simulink model "sim_tase_2025_att_ctrl"  (R2020a)
settings: Solver=ode4  StartTime=0.0  StopTime=30.0  FixedStep=0.01  RelTol=1e-3
values from neighbouring files (symbols this model uses):
  alfa_i_init = zeros(3, NF)    [init_tase_2025_att_ctrl.m]
  beta_ij_init = zeros(3, NF)    [init_tase_2025_att_ctrl.m]
  c1 = 2.5    [init_tase_2025_att_ctrl.m]
  c1_diff_sigma_bar_w = diag([12; 12; 12])    [init_tase_2025_att_ctrl.m]
  c1_diff_ui = diag([25; 30; 20])    [init_tase_2025_att_ctrl.m]
  c2 = 2.0    (= 2)    [init_tase_2025_att_ctrl.m]
  c2_diff_sigma_bar_w = diag([12; 12; 12])    [init_tase_2025_att_ctrl.m]
  c2_diff_ui = diag([50; 50; 10])    [init_tase_2025_att_ctrl.m]
  c3_diff_sigma_bar_w = diag([15; 15; 15])    [init_tase_2025_att_ctrl.m]
  c3_diff_ui = diag([15; 15; 10])    [init_tase_2025_att_ctrl.m]
  dw_aa_t = 0.2 * ones(3, 5) + ( 1.0 - 0.2 ) * rand(3, 5)    [init_tase_2025_att_ctrl.m]
  dw_ff_t = [ 0.4 * ones(1, 5) + ( 1.0 - 0.4 ) * rand(1, 5);                      0.4 * ones(1, 5) + ( 1.0 - 0.4 ) * rand(1, 5);                      0.2 * ones(1, 5) + ( 0.6 - 0.2 ) * rand(1, 5) ]    [init_tase_2025_att_ctrl.m]
  dw_phi_t = ( - pi / 2 ) * ones(3, 5) + ( pi / 2 - ( - pi / 2 ) ) * rand(3, 5)    [init_tase_2025_att_ctrl.m]
  dwci_init = zeros(3,5)    [init_tase_2025_att_ctrl.m]
  err_wi_init = zeros(3, NF)    [init_tase_2025_att_ctrl.m]
  eta_1_ij_init = zeros(3, NF)    [init_tase_2025_att_ctrl.m]
  eta_2_ij_init = zeros(3, NF)    [init_tase_2025_att_ctrl.m]
  h1w = diag([20.0; 20.0; 20.0])    [init_tase_2025_att_ctrl.m]
  h2w = diag([30.0; 35.0; 35.0])    [init_tase_2025_att_ctrl.m]
  h3w = diag([30.0; 25.0; 30.0])    [init_tase_2025_att_ctrl.m]
  Ji = zeros(3,3,NF)    [init_tase_2025_att_ctrl.m]
  k_1_ij_hat_init = zeros(3, NF)    [init_tase_2025_att_ctrl.m]
  k_1_ij_init = zeros(3, NF)    [init_tase_2025_att_ctrl.m]
  k_1_ij_lower = zeros(3, NF)    [init_tase_2025_att_ctrl.m]
  k_1_ij_upper = zeros(3, NF)    [init_tase_2025_att_ctrl.m]
  k_2_ij_init = zeros(3, NF)    [init_tase_2025_att_ctrl.m]
  k_2_ij_lower = zeros(3, NF)    [init_tase_2025_att_ctrl.m]
  k_2_ij_upper = zeros(3, NF)    [init_tase_2025_att_ctrl.m]
  Lamd_diff_sigma_bar_w = 0.8    [init_tase_2025_att_ctrl.m]
  Lamd_diff_ui = 0.8    [init_tase_2025_att_ctrl.m]
  mu1 = 0.2    [init_tase_2025_att_ctrl.m]
  mu2 = 0.2    [init_tase_2025_att_ctrl.m]
  mu_d_w = 100    [init_tase_2025_att_ctrl.m]
  phi_ij_init = ones(3, NF)    [init_tase_2025_att_ctrl.m]
  pos0 = zeros(3, 1)    [init_tase_2025_att_ctrl.m]
  PZ0 = P0(3)    [init_tase_2025_att_ctrl.m]
  PZ1 = 10    [init_tase_2025_att_ctrl.m]
  q_ij_hat_init = zeros(3, NF)    [init_tase_2025_att_ctrl.m]
  Qci_init = repmat([1;0;0;0],1,NF)    [init_tase_2025_att_ctrl.m]
  R0 = 4    [init_tase_2025_att_ctrl.m]
  R1 = 8    [init_tase_2025_att_ctrl.m]
  Rci_init = zeros(3,3,NF)    [init_tase_2025_att_ctrl.m]
  Ri_init = zeros(3,3,NF)    [init_tase_2025_att_ctrl.m]
  Rx2 = 10    [init_tase_2025_att_ctrl.m]
  Ry2 = 6    [init_tase_2025_att_ctrl.m]
  Rz2 = 4    [init_tase_2025_att_ctrl.m]
  T0 = 0    [init_tase_2025_att_ctrl.m]
  T1 = tseq1    (= 10)    [init_tase_2025_att_ctrl.m]
  T2 = tseq1 + tseq12 + tseq2    (= 30)    [init_tase_2025_att_ctrl.m]
  T_ij = repmat([60.0; 60.0; 60.0], 1, NF)    [init_tase_2025_att_ctrl.m]
  ui_init = zeros(3,NF)    [init_tase_2025_att_ctrl.m]
  vel0 = zeros(3, 1)    [init_tase_2025_att_ctrl.m]
  wci_init = zeros(3,5)    [init_tase_2025_att_ctrl.m]
  zeta_diff_sigma_bar_w = 0.3    [init_tase_2025_att_ctrl.m]
  zeta_diff_ui = 0.05    [init_tase_2025_att_ctrl.m]
undefined symbols (not defined in the file or in its folder): cal_frac_squ, p_alfaw1, p_alfaw2, q_alfaw1, q_alfaw2, Qei_init, Qi_init, Rei_init, V_Phi_Rei_init, wei_init, wi_init
(part 5 of 5)

== matlab function sim_tase_2025_att_ctrl/generate angular rate disturbance agent 3 ==
  data: dw_3 output; dw_aa_t input; dw_ff_t input; dw_phi_t input; t input
function dw_3 = fcn(dw_aa_t, dw_ff_t, dw_phi_t, t)
%%%% 姿态动力学方程中的扰动项设置
epsil_t = zeros(3, 1);

for kk = 1:5
    epsil_t = epsil_t + dw_aa_t(:, kk) .* sin( 2 * pi * dw_ff_t(:, kk) * t + dw_phi_t(:, kk) );
end

dw_3 = [ epsil_t(1) + 1.6 * sin( 0.2 * t ) + 2.0 * cos( 0.3 * t ) + 1.4 * sin( 0.5 * t ) ...
                + 4 * exp( -0.1 * t ) * sin( 0.5 * t ) + 3 / ( 1 + exp( -0.2 * ( t - 15 ) ) ); ...
                epsil_t(2) + 1.2 * sin( 0.1 * t ) + 3 * cos( 0.2 * t ) + 0.8 * sin( 0.4 * t ) ...
                + 2 * exp( -0.15 * t ) * cos( 0.6 * t ) + 3 / ( 1 + exp( -0.3 * ( t - 25 ) ) ); ...
                epsil_t(3) + 1.8 * sin( 0.1 * t ) + 1.6 * sin( 0.2 * t ) + 1.6 * cos( 0.3 * t ) ...
                + 4 * exp( -0.05 * t ) * sin( 0.4 * t + pi / 4 ) + 3 / ( 1 + exp( -0.5 * ( t - 20 ) ) ) ];

== matlab function sim_tase_2025_att_ctrl/generate angular rate disturbance agent 4 ==
  data: dw_4 output; dw_aa_t input; dw_ff_t input; dw_phi_t input; t input
function dw_4 = fcn(dw_aa_t, dw_ff_t, dw_phi_t, t)
%%%% 姿态动力学方程中的扰动项设置
epsil_t = zeros(3, 1);

for kk = 1:5
    epsil_t = epsil_t + dw_aa_t(:, kk) .* sin( 2 * pi * dw_ff_t(:, kk) * t + dw_phi_t(:, kk) );
end

dw_4 = [ epsil_t(1) + 1.6 * sin( 0.2 * t ) + 2.0 * cos( 0.3 * t ) + 1.4 * sin( 0.5 * t ) ...
                + 4 * exp( -0.1 * t ) * sin( 0.5 * t ) + 3 / ( 1 + exp( -0.2 * ( t - 15 ) ) ); ...
                epsil_t(2) + 1.2 * sin( 0.1 * t ) + 3 * cos( 0.2 * t ) + 0.8 * sin( 0.4 * t ) ...
                + 2 * exp( -0.15 * t ) * cos( 0.6 * t ) + 3 / ( 1 + exp( -0.3 * ( t - 25 ) ) ); ...
                epsil_t(3) + 1.8 * sin( 0.1 * t ) + 1.6 * sin( 0.2 * t ) + 1.6 * cos( 0.3 * t ) ...
                + 4 * exp( -0.05 * t ) * sin( 0.4 * t + pi / 4 ) + 3 / ( 1 + exp( -0.5 * ( t - 20 ) ) ) ];

== matlab function sim_tase_2025_att_ctrl/generate angular rate disturbance agent 5 ==
  data: dw_5 output; dw_aa_t input; dw_ff_t input; dw_phi_t input; t input
function dw_5 = fcn(dw_aa_t, dw_ff_t, dw_phi_t, t)
%%%% 姿态动力学方程中的扰动项设置
epsil_t = zeros(3, 1);

for kk = 1:5
    epsil_t = epsil_t + dw_aa_t(:, kk) .* sin( 2 * pi * dw_ff_t(:, kk) * t + dw_phi_t(:, kk) );
end

dw_5 = [ epsil_t(1) + 1.6 * sin( 0.2 * t ) + 2.0 * cos( 0.3 * t ) + 1.4 * sin( 0.5 * t ) ...
                + 4 * exp( -0.1 * t ) * sin( 0.5 * t ) + 3 / ( 1 + exp( -0.2 * ( t - 15 ) ) ); ...
                epsil_t(2) + 1.2 * sin( 0.1 * t ) + 3 * cos( 0.2 * t ) + 0.8 * sin( 0.4 * t ) ...
                + 2 * exp( -0.15 * t ) * cos( 0.6 * t ) + 3 / ( 1 + exp( -0.3 * ( t - 25 ) ) ); ...
                epsil_t(3) + 1.8 * sin( 0.1 * t ) + 1.6 * sin( 0.2 * t ) + 1.6 * cos( 0.3 * t ) ...
                + 4 * exp( -0.05 * t ) * sin( 0.4 * t + pi / 4 ) + 3 / ( 1 + exp( -0.5 * ( t - 20 ) ) ) ];

== matlab function sim_tase_2025_att_ctrl/combine norminal formation control input ==
  data: ui_1 input; ui_vec output; ui_2 input; ui_3 input; ui_4 input; ui_5 input
function ui_vec = fcn(ui_1, ui_2, ui_3, ui_4, ui_5)
%%%% 合并领导者编队跟踪误差结果
ui_vec = [ui_1(:), ui_2(:), ui_3(:), ui_4(:), ui_5(:)];

== matlab function sim_tase_2025_att_ctrl/control input generator agent 1 ==
  data: u0 input; ui output
function ui  = fcn(u0)
%%%% 给出领导者参考加速度控制输入
g0 = 9.80663;
e3 = [0;0;1];

ui = g0 * e3 + u0(:);

== matlab function sim_tase_2025_att_ctrl/control input generator agent 2 ==
  data: u0 input; ui output
function ui  = fcn(u0)
%%%% 给出领导者参考加速度控制输入
g0 = 9.80663;
e3 = [0;0;1];

ui = g0 * e3 + u0(:);

== matlab function sim_tase_2025_att_ctrl/control input generator agent 3 ==
  data: u0 input; ui output
function ui  = fcn(u0)
%%%% 给出领导者参考加速度控制输入
g0 = 9.80663;
e3 = [0;0;1];

ui = g0 * e3 + u0(:);

== matlab function sim_tase_2025_att_ctrl/control input generator agent 4 ==
  data: u0 input; ui output
function ui  = fcn(u0)
%%%% 给出领导者参考加速度控制输入
g0 = 9.80663;
e3 = [0;0;1];

ui = g0 * e3 + u0(:);

== matlab function sim_tase_2025_att_ctrl/combine k_1_ij_hat ==
  data: k_1_ij_hat_node_1 input; k_1_ij_hat_vec output; k_1_ij_hat_node_2 input; k_1_ij_hat_node_3 input; k_1_ij_hat_node_4 input; k_1_ij_hat_node_5 input
function k_1_ij_hat_vec = fcn(k_1_ij_hat_node_1, k_1_ij_hat_node_2, k_1_ij_hat_node_3, k_1_ij_hat_node_4, k_1_ij_hat_node_5)
%%%% 合并预设性能函数
k_1_ij_hat_vec = [k_1_ij_hat_node_1(:), k_1_ij_hat_node_2(:), k_1_ij_hat_node_3(:), k_1_ij_hat_node_4(:), k_1_ij_hat_node_5(:)];

== matlab function sim_tase_2025_att_ctrl/control input generator agent 5 ==
  data: u0 input; ui output
function ui  = fcn(u0)
%%%% 给出领导者参考加速度控制输入
g0 = 9.80663;
e3 = [0;0;1];

ui = g0 * e3 + u0(:);

== matlab function sim_tase_2025_att_ctrl/cal q_ij_hat agent 1 ==
  data: k_1_ij_lower input; q_ij_hat_node_1 output; k_1_ij_vec input; Qi_vec input
function q_ij_hat_node_1 = fcn(k_1_ij_lower, k_1_ij_vec, Qi_vec)
%%%% 计算用于消除超调的四元数
iiuav = 1;
q_ij_hat_node_1 = zeros(3,1);
for jj = 1:3
    if Qi_vec(jj + 1, iiuav) >= 0
        q_ij_hat_node_1(jj) = Qi_vec(jj + 1, iiuav) - (1/2) * ( k_1_ij_vec(jj,iiuav) - k_1_ij_lower(jj,iiuav) );
    else
        q_ij_hat_node_1(jj) = Qi_vec(jj + 1, iiuav) - (1/2) * ( k_1_ij_lower(jj,iiuav) - k_1_ij_vec(jj,iiuav) );
    end
end

== matlab function sim_tase_2025_att_ctrl/cal q_ij_hat agent 2 ==
  data: k_1_ij_lower input; q_ij_hat_node_2 output; k_1_ij_vec input; Qi_vec input
function q_ij_hat_node_2 = fcn(k_1_ij_lower, k_1_ij_vec, Qi_vec)
%%%% 计算用于消除超调的四元数
iiuav = 2;
q_ij_hat_node_2 = zeros(3,1);
for jj = 1:3
    if Qi_vec(jj + 1, iiuav) >= 0
        q_ij_hat_node_2(jj) = Qi_vec(jj + 1, iiuav) - (1/2) * ( k_1_ij_vec(jj,iiuav) - k_1_ij_lower(jj,iiuav) );
    else
        q_ij_hat_node_2(jj) = Qi_vec(jj + 1, iiuav) - (1/2) * ( k_1_ij_lower(jj,iiuav) - k_1_ij_vec(jj,iiuav) );
    end
end

== matlab function sim_tase_2025_att_ctrl/cal q_ij_hat agent 3 ==
  data: k_1_ij_lower input; q_ij_hat_node_3 output; k_1_ij_vec input; Qi_vec input
function q_ij_hat_node_3 = fcn(k_1_ij_lower, k_1_ij_vec, Qi_vec)
%%%% 计算用于消除超调的四元数
iiuav = 3;
q_ij_hat_node_3 = zeros(3,1);
for jj = 1:3
    if Qi_vec(jj + 1, iiuav) >= 0
        q_ij_hat_node_3(jj) = Qi_vec(jj + 1, iiuav) - (1/2) * ( k_1_ij_vec(jj,iiuav) - k_1_ij_lower(jj,iiuav) );
    else
        q_ij_hat_node_3(jj) = Qi_vec(jj + 1, iiuav) - (1/2) * ( k_1_ij_lower(jj,iiuav) - k_1_ij_vec(jj,iiuav) );
    end
end

== matlab function sim_tase_2025_att_ctrl/cal q_ij_hat agent 4 ==
  data: k_1_ij_lower input; q_ij_hat_node_4 output; k_1_ij_vec input; Qi_vec input
function q_ij_hat_node_4 = fcn(k_1_ij_lower, k_1_ij_vec, Qi_vec)
%%%% 计算用于消除超调的四元数
iiuav = 4;
q_ij_hat_node_4 = zeros(3,1);
for jj = 1:3
    if Qi_vec(jj + 1, iiuav) >= 0
        q_ij_hat_node_4(jj) = Qi_vec(jj + 1, iiuav) - (1/2) * ( k_1_ij_vec(jj,iiuav) - k_1_ij_lower(jj,iiuav) );
    else
        q_ij_hat_node_4(jj) = Qi_vec(jj + 1, iiuav) - (1/2) * ( k_1_ij_lower(jj,iiuav) - k_1_ij_vec(jj,iiuav) );
    end
end

== matlab function sim_tase_2025_att_ctrl/cal q_ij_hat agent 5 ==
  data: k_1_ij_lower input; q_ij_hat_node_5 output; k_1_ij_vec input; Qi_vec input
function q_ij_hat_node_5 = fcn(k_1_ij_lower, k_1_ij_vec, Qi_vec)
%%%% 计算用于消除超调的四元数
iiuav = 5;
q_ij_hat_node_5 = zeros(3,1);
for jj = 1:3
    if Qi_vec(jj + 1, iiuav) >= 0
        q_ij_hat_node_5(jj) = Qi_vec(jj + 1, iiuav) - (1/2) * ( k_1_ij_vec(jj,iiuav) - k_1_ij_lower(jj,iiuav) );
    else
        q_ij_hat_node_5(jj) = Qi_vec(jj + 1, iiuav) - (1/2) * ( k_1_ij_lower(jj,iiuav) - k_1_ij_vec(jj,iiuav) );
    end
end

== matlab function sim_tase_2025_att_ctrl/cal d_theta_hat ==
  data: c1 input; d_ui_hat output; d_dui_hat output; d_d2ui_hat output; c2 input; c3 input; chi_t input; ui_sig_1 input; ui_sig_2 input; ui_sig_3 input; ui_sig_4 input; ui_sig_5 input; ui_sig_6 input; dui_hat input; d2ui_hat input
function [d_ui_hat, d_dui_hat, d_d2ui_hat] = fcn(c1, c2, c3, chi_t, ui_sig_1, ui_sig_2, ui_sig_3, ...
                                                                                        ui_sig_4, ui_sig_5, ui_sig_6, dui_hat, d2ui_hat)
d_d2ui_hat = -chi_t .* c1 * ui_sig_1(:) - (1 - chi_t) .* c1 * ui_sig_2(:);
d_dui_hat = -chi_t .* c2 * ui_sig_3(:) - (1 - chi_t) .* c2 * ui_sig_4(:) + d2ui_hat(:);
d_ui_hat = -chi_t .* c3 * ui_sig_5(:) - (1 - chi_t) .* c3 * ui_sig_6(:) + dui_hat(:);

== matlab function sim_tase_2025_att_ctrl/combine q_ij_hat ==
  data: q_ij_hat_node_1 input; q_ij_hat_vec output; q_ij_hat_node_2 input; q_ij_hat_node_3 input; q_ij_hat_node_4 input; q_ij_hat_node_5 input
function q_ij_hat_vec = fcn(q_ij_hat_node_1, q_ij_hat_node_2, q_ij_hat_node_3, q_ij_hat_node_4, q_ij_hat_node_5)
%%%% 合并用于消除超调的四元数
q_ij_hat_vec = [q_ij_hat_node_1(:), q_ij_hat_node_2(:), q_ij_hat_node_3(:), q_ij_hat_node_4(:), q_ij_hat_node_5(:)];

== matlab function sim_tase_2025_att_ctrl/cal eta_1_ij agent 1 ==
  data: Qi_vec input; eta_1_ij_node_1 output; k_1_ij_vec input
function eta_1_ij_node_1 = fcn(Qi_vec, k_1_ij_vec)
%%%% 计算障碍函数
iiuav = 1;
eta_1_ij_node_1 = zeros(3,1);
for jj = 1:3
    eta_1_ij_node_1(jj) = tan( (pi/2) * ( Qi_vec(jj + 1, iiuav) / k_1_ij_vec(jj, iiuav) ) );
end

== matlab function sim_tase_2025_att_ctrl/cal eta_1_ij agent 2 ==
  data: Qi_vec input; eta_1_ij_node_2 output; k_1_ij_vec input
function eta_1_ij_node_2 = fcn(Qi_vec, k_1_ij_vec)
%%%% 计算障碍函数
iiuav = 2;
eta_1_ij_node_2 = zeros(3,1);
for jj = 1:3
    eta_1_ij_node_2(jj) = tan( (pi/2) * ( Qi_vec(jj + 1, iiuav) / k_1_ij_vec(jj, iiuav) ) );
end

== matlab function sim_tase_2025_att_ctrl/cal eta_1_ij agent 3 ==
  data: Qi_vec input; eta_1_ij_node_3 output; k_1_ij_vec input
function eta_1_ij_node_3 = fcn(Qi_vec, k_1_ij_vec)
%%%% 计算障碍函数
iiuav = 3;
eta_1_ij_node_3 = zeros(3,1);
for jj = 1:3
    eta_1_ij_node_3(jj) = tan( (pi/2) * ( Qi_vec(jj + 1, iiuav) / k_1_ij_vec(jj, iiuav) ) );
end

== matlab function sim_tase_2025_att_ctrl/combine eta_1_ij ==
  data: eta_1_ij_node_1 input; eta_1_ij_vec output; eta_1_ij_node_2 input; eta_1_ij_node_3 input; eta_1_ij_node_4 input; eta_1_ij_node_5 input
function eta_1_ij_vec = fcn(eta_1_ij_node_1, eta_1_ij_node_2, eta_1_ij_node_3, eta_1_ij_node_4, eta_1_ij_node_5)
%%%% 合并预设性能函数
eta_1_ij_vec = [eta_1_ij_node_1(:), eta_1_ij_node_2(:), eta_1_ij_node_3(:), eta_1_ij_node_4(:), eta_1_ij_node_5(:)];

== matlab function sim_tase_2025_att_ctrl/cal eta_1_ij agent 4 ==
  data: Qi_vec input; eta_1_ij_node_4 output; k_1_ij_vec input
function eta_1_ij_node_4 = fcn(Qi_vec, k_1_ij_vec)
%%%% 计算障碍函数
iiuav = 4;
eta_1_ij_node_4 = zeros(3,1);
for jj = 1:3
    eta_1_ij_node_4(jj) = tan( (pi/2) * ( Qi_vec(jj + 1, iiuav) / k_1_ij_vec(jj, iiuav) ) );
end

== matlab function sim_tase_2025_att_ctrl/cal sig ==
  data: x input; z output; y input
function z = fcn(x, y)
z = x(:) .* sign(y(:));

== matlab function sim_tase_2025_att_ctrl/cal sig1 ==
  data: x input; z output; y input
function z = fcn(x, y)
z = x(:) .* sign(y(:));

== matlab function sim_tase_2025_att_ctrl/cal sig2 ==
  data: x input; z output; y input
function z = fcn(x, y)
z = x(:) .* sign(y(:));

== matlab function sim_tase_2025_att_ctrl/cal sig3 ==
  data: x input; z output; y input
function z = fcn(x, y)
z = x(:) .* sign(y(:));

== matlab function sim_tase_2025_att_ctrl/cal sig4 ==
  data: x input; z output; y input
function z = fcn(x, y)
z = x(:) .* sign(y(:));

== matlab function sim_tase_2025_att_ctrl/cal sig5 ==
  data: x input; z output; y input
function z = fcn(x, y)
z = x(:) .* sign(y(:));

== matlab function sim_tase_2025_att_ctrl/trans to column10 ==
  data: x input; y output
function y = fcn(x)
y = x(:);

== matlab function sim_tase_2025_att_ctrl/trans to column5 ==
  data: x input; y output
function y = fcn(x)
y = x(:);

== matlab function sim_tase_2025_att_ctrl/trans to column6 ==
  data: x input; y output
function y = fcn(x)
y = x(:);

== matlab function sim_tase_2025_att_ctrl/trans to column7 ==
  data: x input; y output
function y = fcn(x)
y = x(:);

== matlab function sim_tase_2025_att_ctrl/trans to column8 ==
  data: x input; y output
function y = fcn(x)
y = x(:);

== matlab function sim_tase_2025_att_ctrl/trans to column9 ==
  data: x input; y output
function y = fcn(x)
y = x(:);

== matlab function sim_tase_2025_att_ctrl/choose ui agent 1 ==
  data: x input; y output
function y = fcn(x)
iiuav = 1;
y = x(:,iiuav);

== matlab function sim_tase_2025_att_ctrl/cal d_theta_hat1 ==
  data: c1 input; d_ui_hat output; d_dui_hat output; d_d2ui_hat output; c2 input; c3 input; chi_t input; ui_sig_1 input; ui_sig_2 input; ui_sig_3 input; ui_sig_4 input; ui_sig_5 input; ui_sig_6 input; dui_hat input; d2ui_hat input
function [d_ui_hat, d_dui_hat, d_d2ui_hat] = fcn(c1, c2, c3, chi_t, ui_sig_1, ui_sig_2, ui_sig_3, ...
                                                                                        ui_sig_4, ui_sig_5, ui_sig_6, dui_hat, d2ui_hat)
d_d2ui_hat = -chi_t .* c1 * ui_sig_1(:) - (1 - chi_t) .* c1 * ui_sig_2(:);
d_dui_hat = -chi_t .* c2 * ui_sig_3(:) - (1 - chi_t) .* c2 * ui_sig_4(:) + d2ui_hat(:);
d_ui_hat = -chi_t .* c3 * ui_sig_5(:) - (1 - chi_t) .* c3 * ui_sig_6(:) + dui_hat(:);

== matlab function sim_tase_2025_att_ctrl/cal sig10 ==
  data: x input; z output; y input
function z = fcn(x, y)
z = x(:) .* sign(y(:));

== matlab function sim_tase_2025_att_ctrl/cal sig11 ==
  data: x input; z output; y input
function z = fcn(x, y)
z = x(:) .* sign(y(:));

== matlab function sim_tase_2025_att_ctrl/cal sig6 ==
  data: x input; z output; y input
function z = fcn(x, y)
z = x(:) .* sign(y(:));

== matlab function sim_tase_2025_att_ctrl/cal sig7 ==
  data: x input; z output; y input
function z = fcn(x, y)
z = x(:) .* sign(y(:));

== matlab function sim_tase_2025_att_ctrl/cal sig8 ==
  data: x input; z output; y input
function z = fcn(x, y)
z = x(:) .* sign(y(:));

== matlab function sim_tase_2025_att_ctrl/cal sig9 ==
  data: x input; z output; y input
function z = fcn(x, y)
z = x(:) .* sign(y(:));

== matlab function sim_tase_2025_att_ctrl/choose ui agent 2 ==
  data: x input; y output
function y = fcn(x)
iiuav = 2;
y = x(:,iiuav);

== matlab function sim_tase_2025_att_ctrl/trans to column11 ==
  data: x input; y output
function y = fcn(x)
y = x(:);

== matlab function sim_tase_2025_att_ctrl/trans to column12 ==
  data: x input; y output
function y = fcn(x)
y = x(:);

== matlab function sim_tase_2025_att_ctrl/trans to column13 ==
  data: x input; y output
function y = fcn(x)
y = x(:);

== matlab function sim_tase_2025_att_ctrl/trans to column14 ==
  data: x input; y output
function y = fcn(x)
y = x(:);

== matlab function sim_tase_2025_att_ctrl/trans to column15 ==
  data: x input; y output
function y = fcn(x)
y = x(:);

== matlab function sim_tase_2025_att_ctrl/trans to column16 ==
  data: x input; y output
function y = fcn(x)
y = x(:);

== matlab function sim_tase_2025_att_ctrl/cal d_theta_hat2 ==
  data: c1 input; d_ui_hat output; d_dui_hat output; d_d2ui_hat output; c2 input; c3 input; chi_t input; ui_sig_1 input; ui_sig_2 input; ui_sig_3 input; ui_sig_4 input; ui_sig_5 input; ui_sig_6 input; dui_hat input; d2ui_hat input
function [d_ui_hat, d_dui_hat, d_d2ui_hat] = fcn(c1, c2, c3, chi_t, ui_sig_1, ui_sig_2, ui_sig_3, ...
                                                                                        ui_sig_4, ui_sig_5, ui_sig_6, dui_hat, d2ui_hat)
d_d2ui_hat = -chi_t .* c1 * ui_sig_1(:) - (1 - chi_t) .* c1 * ui_sig_2(:);
d_dui_hat = -chi_t .* c2 * ui_sig_3(:) - (1 - chi_t) .* c2 * ui_sig_4(:) + d2ui_hat(:);
d_ui_hat = -chi_t .* c3 * ui_sig_5(:) - (1 - chi_t) .* c3 * ui_sig_6(:) + dui_hat(:);

== matlab function sim_tase_2025_att_ctrl/cal sig12 ==
  data: x input; z output; y input
function z = fcn(x, y)
z = x(:) .* sign(y(:));

== matlab function sim_tase_2025_att_ctrl/cal sig13 ==
  data: x input; z output; y input
function z = fcn(x, y)
z = x(:) .* sign(y(:));

== matlab function sim_tase_2025_att_ctrl/cal sig14 ==
  data: x input; z output; y input
function z = fcn(x, y)
z = x(:) .* sign(y(:));

== matlab function sim_tase_2025_att_ctrl/cal sig15 ==
  data: x input; z output; y input
function z = fcn(x, y)
z = x(:) .* sign(y(:));

== matlab function sim_tase_2025_att_ctrl/cal sig16 ==
  data: x input; z output; y input
function z = fcn(x, y)
z = x(:) .* sign(y(:));

== matlab function sim_tase_2025_att_ctrl/cal sig17 ==
  data: x input; z output; y input
function z = fcn(x, y)
z = x(:) .* sign(y(:));

== matlab function sim_tase_2025_att_ctrl/choose ui agent 3 ==
  data: x input; y output
function y = fcn(x)
iiuav = 3;
y = x(:,iiuav);

== matlab function sim_tase_2025_att_ctrl/trans to column17 ==
  data: x input; y output
function y = fcn(x)
y = x(:);

== matlab function sim_tase_2025_att_ctrl/trans to column18 ==
  data: x input; y output
function y = fcn(x)
y = x(:);

== matlab function sim_tase_2025_att_ctrl/trans to column19 ==
  data: x input; y output
function y = fcn(x)
y = x(:);

== matlab function sim_tase_2025_att_ctrl/trans to column20 ==
  data: x input; y output
function y = fcn(x)
y = x(:);

== matlab function sim_tase_2025_att_ctrl/trans to column21 ==
  data: x input; y output
function y = fcn(x)
y = x(:);

== matlab function sim_tase_2025_att_ctrl/trans to column22 ==
  data: x input; y output
function y = fcn(x)
y = x(:);

== matlab function sim_tase_2025_att_ctrl/cal d_theta_hat3 ==
  data: c1 input; d_ui_hat output; d_dui_hat output; d_d2ui_hat output; c2 input; c3 input; chi_t input; ui_sig_1 input; ui_sig_2 input; ui_sig_3 input; ui_sig_4 input; ui_sig_5 input; ui_sig_6 input; dui_hat input; d2ui_hat input
function [d_ui_hat, d_dui_hat, d_d2ui_hat] = fcn(c1, c2, c3, chi_t, ui_sig_1, ui_sig_2, ui_sig_3, ...
                                                                                        ui_sig_4, ui_sig_5, ui_sig_6, dui_hat, d2ui_hat)
d_d2ui_hat = -chi_t .* c1 * ui_sig_1(:) - (1 - chi_t) .* c1 * ui_sig_2(:);
d_dui_hat = -chi_t .* c2 * ui_sig_3(:) - (1 - chi_t) .* c2 * ui_sig_4(:) + d2ui_hat(:);
d_ui_hat = -chi_t .* c3 * ui_sig_5(:) - (1 - chi_t) .* c3 * ui_sig_6(:) + dui_hat(:);

== matlab function sim_tase_2025_att_ctrl/cal sig18 ==
  data: x input; z output; y input
function z = fcn(x, y)
z = x(:) .* sign(y(:));

== matlab function sim_tase_2025_att_ctrl/cal eta_1_ij agent 5 ==
  data: Qi_vec input; eta_1_ij_node_5 output; k_1_ij_vec input
function eta_1_ij_node_5 = fcn(Qi_vec, k_1_ij_vec)
%%%% 计算障碍函数
iiuav = 5;
eta_1_ij_node_5 = zeros(3,1);
for jj = 1:3
    eta_1_ij_node_5(jj) = tan( (pi/2) * ( Qi_vec(jj + 1, iiuav) / k_1_ij_vec(jj, iiuav) ) );
end

== matlab function sim_tase_2025_att_ctrl/cal sig19 ==
  data: x input; z output; y input
function z = fcn(x, y)
z = x(:) .* sign(y(:));

== matlab function sim_tase_2025_att_ctrl/cal sig20 ==
  data: x input; z output; y input
function z = fcn(x, y)
z = x(:) .* sign(y(:));

== matlab function sim_tase_2025_att_ctrl/cal sig21 ==
  data: x input; z output; y input
function z = fcn(x, y)
z = x(:) .* sign(y(:));

== matlab function sim_tase_2025_att_ctrl/process velocity ==
  data: T0 input; T1 input; T2 input; PZ0 input; PZ1 input; R0 input; R1 input; Rx2 input; Ry2 input; Rz2 input; t input; V_init_out output
function V_init_out = fcn(T0, T1, T2, PZ0, PZ1, R0, R1, Rx2, Ry2, Rz2, t)
V_init_out = zeros(3, 1);
if t < T1 + 1e-05
    V_init_out(1, 1) = ( cos( ( 2 * pi * ( t - T0 ) ) / ( T0 - T1 ) ) * ( R0 - R1 ) ) / ( T0 - T1 ) ...
                                    - ( 2 * pi * sin( ( 2 * pi * ( t - T0 ) ) / ( T0 - T1 ) ) * ( R0 + ( ( R0 - R1 ) * ( t - T0 ) ) / ( T0 - T1 ) ) ) / ( T0 - T1 );
    V_init_out(2, 1) = ( sin( ( 2 * pi * ( t - T0 ) ) / ( T0 - T1 ) ) * ( R0 - R1 ) ) / ( T0 - T1 ) ...
                                    + ( 2 * pi * cos( ( 2 * pi * ( t - T0 ) ) / ( T0 - T1 ) ) * ( R0 + ( ( R0 - R1 ) * ( t - T0 ) ) / ( T0 - T1 ) ) ) / ( T0 - T1 );
    V_init_out(3, 1) = ( PZ0 - PZ1 ) / ( T0 - T1 );
else
    V_init_out(1, 1) = ( 2 * Rx2 * pi * sin( ( 2 * pi * ( t - T1 ) ) / ( T1 - T2 ) ) ) / ( T1 - T2 );
    V_init_out(2, 1) = ( 4 * Ry2 * pi * cos( ( 4 * pi * ( t - T1 ) ) / ( T1 - T2 ) ) ) / ( T1 - T2 );
    V_init_out(3, 1) = - ( 4 * Rz2 * pi * cos( ( 4 * pi * ( t - T1 ) ) / ( T1 - T2 ) ) ) / ( T1 - T2 );
end

== matlab function sim_tase_2025_att_ctrl/cal sig22 ==
  data: x input; z output; y input
function z = fcn(x, y)
z = x(:) .* sign(y(:));

== matlab function sim_tase_2025_att_ctrl/cal sig23 ==
  data: x input; z output; y input
function z = fcn(x, y)
z = x(:) .* sign(y(:));

== matlab function sim_tase_2025_att_ctrl/choose ui agent 4 ==
  data: x input; y output
function y = fcn(x)
iiuav = 4;
y = x(:,iiuav);

== matlab function sim_tase_2025_att_ctrl/trans to column23 ==
  data: x input; y output
function y = fcn(x)
y = x(:);

== matlab function sim_tase_2025_att_ctrl/trans to column24 ==
  data: x input; y output
function y = fcn(x)
y = x(:);

== matlab function sim_tase_2025_att_ctrl/trans to column25 ==
  data: x input; y output
function y = fcn(x)
y = x(:);

== matlab function sim_tase_2025_att_ctrl/trans to column26 ==
  data: x input; y output
function y = fcn(x)
y = x(:);

== matlab function sim_tase_2025_att_ctrl/trans to column27 ==
  data: x input; y output
function y = fcn(x)
y = x(:);

== matlab function sim_tase_2025_att_ctrl/trans to column28 ==
  data: x input; y output
function y = fcn(x)
y = x(:);

== matlab function sim_tase_2025_att_ctrl/cal d_theta_hat4 ==
  data: c1 input; d_ui_hat output; d_dui_hat output; d_d2ui_hat output; c2 input; c3 input; chi_t input; ui_sig_1 input; ui_sig_2 input; ui_sig_3 input; ui_sig_4 input; ui_sig_5 input; ui_sig_6 input; dui_hat input; d2ui_hat input
function [d_ui_hat, d_dui_hat, d_d2ui_hat] = fcn(c1, c2, c3, chi_t, ui_sig_1, ui_sig_2, ui_sig_3, ...
                                                                                        ui_sig_4, ui_sig_5, ui_sig_6, dui_hat, d2ui_hat)
d_d2ui_hat = -chi_t .* c1 * ui_sig_1(:) - (1 - chi_t) .* c1 * ui_sig_2(:);
d_dui_hat = -chi_t .* c2 * ui_sig_3(:) - (1 - chi_t) .* c2 * ui_sig_4(:) + d2ui_hat(:);
d_ui_hat = -chi_t .* c3 * ui_sig_5(:) - (1 - chi_t) .* c3 * ui_sig_6(:) + dui_hat(:);

== matlab function sim_tase_2025_att_ctrl/cal sig24 ==
  data: x input; z output; y input
function z = fcn(x, y)
z = x(:) .* sign(y(:));

== matlab function sim_tase_2025_att_ctrl/cal sig25 ==
  data: x input; z output; y input
function z = fcn(x, y)
z = x(:) .* sign(y(:));

== matlab function sim_tase_2025_att_ctrl/cal sig26 ==
  data: x input; z output; y input
function z = fcn(x, y)
z = x(:) .* sign(y(:));

== matlab function sim_tase_2025_att_ctrl/cal sig27 ==
  data: x input; z output; y input
function z = fcn(x, y)
z = x(:) .* sign(y(:));

== matlab function sim_tase_2025_att_ctrl/cal sig28 ==
  data: x input; z output; y input
function z = fcn(x, y)
z = x(:) .* sign(y(:));

== matlab function sim_tase_2025_att_ctrl/cal sig29 ==
  data: x input; z output; y input
function z = fcn(x, y)
z = x(:) .* sign(y(:));

== matlab function sim_tase_2025_att_ctrl/choose ui agent 5 ==
  data: x input; y output
function y = fcn(x)
iiuav = 5;
y = x(:,iiuav);
